simulink model "FPLQR"  (R2025a)
settings: Solver=VariableStepAuto  StartTime=0.0  StopTime=0.5  MaxStep=0.0001  RelTol=1e-3
settings Model: Creator=Faheem  LastModifiedBy=Faheem

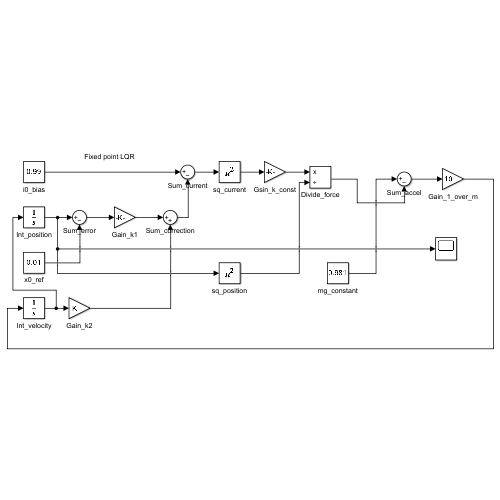
[thumbnail: Simulink's stored preview of the top-level diagram]
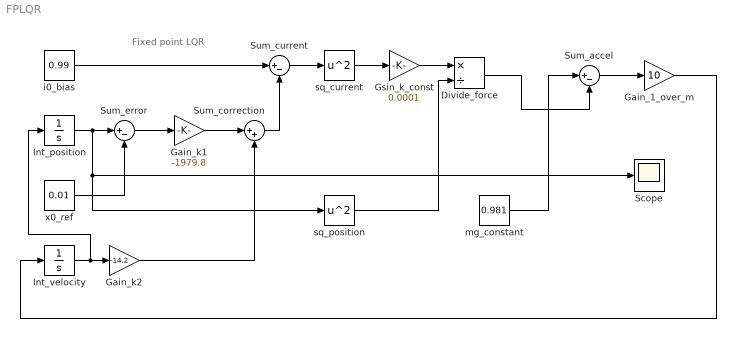
== system FPLQR ==
  note: Fixed point LQR
  Divide_force : Product  Inputs=*/
  Gain_1_over_m : Gain  Gain=10
  Gain_k1 : Gain  Gain=-1979.8
  Gain_k2 : Gain  Gain=-14.2
  Gsin_k_const : Gain  Gain=0.0001
  Int_position : Integrator  InitialCondition=0.0101
  Int_velocity : Integrator
  Scope : Scope
      settings: ActiveDisplayYMinimum=0.00994744564351164  ActiveDisplayYMaximum=0.010143608483841758
  Sum_accel : Sum  Inputs=|+-
  Sum_correction : Sum  Inputs=|++
  Sum_current : Sum  Inputs=|+-
  Sum_error : Sum  Inputs=|+-
  i0_bias : Constant  Value=0.99
  mg_constant : Constant  Value=0.981
  sq_current : Math  Operator=square
  sq_position : Math  Operator=square
  x0_ref : Constant  Value=0.01
  wires:
  Int_position/1 -> Scope/1, sq_position/1, Sum_error/1
  x0_ref/1 -> Sum_error/2
  Sum_error/1 -> Gain_k1/1
  Int_velocity/1 -> Int_position/1, Gain_k2/1
  Gain_k1/1 -> Sum_correction/1
  Gain_k2/1 -> Sum_correction/2
  i0_bias/1 -> Sum_current/1
  Sum_correction/1 -> Sum_current/2
  Sum_current/1 -> sq_current/1
  sq_current/1 -> Gsin_k_const/1
  Gsin_k_const/1 -> Divide_force/1
  sq_position/1 -> Divide_force/2
  mg_constant/1 -> Sum_accel/1
  Divide_force/1 -> Sum_accel/2
  Sum_accel/1 -> Gain_1_over_m/1
  Gain_1_over_m/1 -> Int_velocity/1
